simulink model "chap4_8"  (Simulink 3.00)
settings: Solver=ode45  StartTime=0.0  StopTime=1  RelTol=1e-3
undefined symbols (not defined in the file or in its folder): chap4_8m1, chap4_8m2
libraries: simulink3 x1

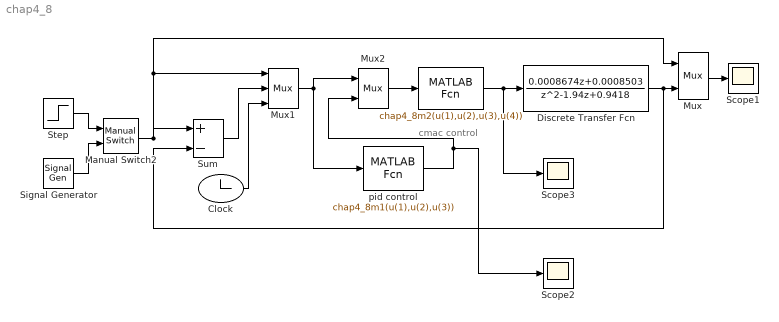
== system chap4_8 ==
  note: cmac control
  "    " : MATLABFcn  MATLABFcn=chap4_8m2(u(1),u(2),u(3),u(4))  OutputWidth=1  OutputSignalType=auto
  "    pid control" : MATLABFcn  MATLABFcn=chap4_8m1(u(1),u(2),u(3))  OutputWidth=1  OutputSignalType=auto
  Clock : Clock
      settings: Decimation=10
  Discrete Transfer Fcn : DiscreteTransferFcn  Numerator=[0.0008674 0.0008503]  Denominator=[1 -1.94 0.9418]  SampleTime=0.001
  Manual Switch2 : simulink3/Nonlinear/Manual Switch  sw=0  action=0
  Mux : Mux  Inputs=2
      settings: DisplayOption=none
  Mux1 : Mux  Inputs=3
      settings: DisplayOption=none
  Mux2 : Mux  Inputs=2
      settings: DisplayOption=none
  Scope1 : Scope
      settings: TimeRange=0.2  YMin=0.988  YMax=1  SaveToWorkspace=off  SaveName=ScopeData  MaxRows=50000  Decimation=0.001  SampleInput=on  SampleTime=0.001
  Scope2 : Scope
      settings: TimeRange=0.2  YMin=-0.00045  YMax=-0.0004225  SaveToWorkspace=off  SaveName=ScopeData  MaxRows=50000  Decimation=0.001  SampleInput=on  SampleTime=0.001
  Scope3 : Scope
      settings: TimeRange=0.2  YMin=0.52382  YMax=0.523925  SaveToWorkspace=off  SaveName=ScopeData  MaxRows=50000  Decimation=0.001  SampleInput=on  SampleTime=0.001
  Signal Generator : SignalGenerator  WaveForm=square  Amplitude=0.5  Frequency=4  Units=Hertz
  Step : Step  Time=0  Before=0  After=1  SampleTime=0.001
  Sum : Sum  Inputs=|+-  SaturateOnIntegerOverflow=on
  wires:
  Sum/1 -> Mux1/2
  Mux/1 -> Scope1/1
  Clock/1 -> Mux1/3
  Mux1/1 -> "    pid control"/1, Mux2/1
  Mux2/1 -> "    "/1
  Manual Switch2/1 -> Sum/1, Mux1/1, Mux/1
  "    pid control"/1 -> Mux2/2, Scope2/1
  Discrete Transfer Fcn/1 -> Sum/2, Mux/2
  Step/1 -> Manual Switch2/1
  Signal Generator/1 -> Manual Switch2/2
  "    "/1 -> Scope3/1, Discrete Transfer Fcn/1
